simulink model "test_motor"  (R2015b)
settings: Solver=VariableStepAuto  StartTime=0.0  StopTime=10.0  RelTol=1e-3
libraries: simulink x1
settings Model: Creator=Deepak  LastModifiedBy=Deepak

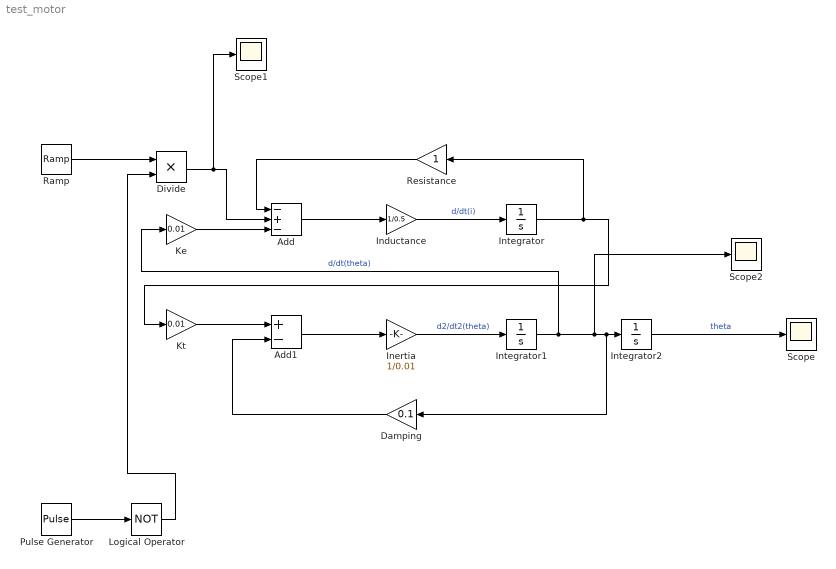
== system test_motor ==
  Add : Sum  Inputs=-+-
  Add1 : Sum  Inputs=+-
  Damping : Gain  Gain=0.1
  Divide : Product  Inputs=**
  Inductance : Gain  Gain=1/0.5
  Inertia : Gain  Gain=1/0.01
  Integrator : Integrator
  Integrator1 : Integrator
  Integrator2 : Integrator
  Ke : Gain  Gain=0.01
  Kt : Gain  Gain=0.01
  Logical Operator : Logic  Operator=NOT  AllPortsSameDT=off  OutDataTypeStr=boolean
  Pulse Generator : DiscretePulseGenerator  PulseType=Time based  Period=10  PulseWidth=50  PhaseDelay=5
  Ramp : simulink/Sources/Ramp  slope=1  start=0  X0=0
  Resistance : Gain
  Scope : Scope
  Scope1 : Scope
  Scope2 : Scope
  wires:
  Resistance/1 -> Add/1
  Ke/1 -> Add/3
  Add/1 -> Inductance/1
  Inductance/1 -> Integrator/1  "d/dt(i)"
  Kt/1 -> Add1/1
  Add1/1 -> Inertia/1
  Inertia/1 -> Integrator1/1  "d2/dt2(theta)"
  Integrator1/1 -> Scope2/1, Damping/1, Integrator2/1, Ke/1  "d/dt(theta)"
  Integrator2/1 -> Scope/1  "theta"
  Integrator/1 -> Resistance/1, Kt/1
  Damping/1 -> Add1/2
  Pulse Generator/1 -> Logical Operator/1
  Ramp/1 -> Divide/1
  Divide/1 -> Scope1/1, Add/2
  Logical Operator/1 -> Divide/2
